simulink model "flightControl"  (R2024a)
settings: Solver=VariableStepAuto  StartTime=0.0  StopTime=25  RelTol=1e-3
settings Model: Creator=Tamir Azaouag  LastModifiedBy=Tamir Azaouag

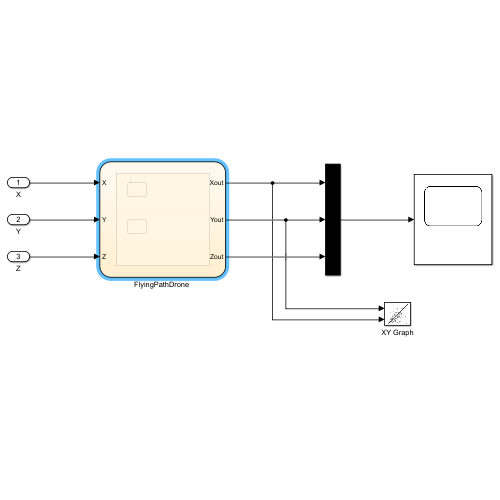
[thumbnail: Simulink's stored preview of the top-level diagram]
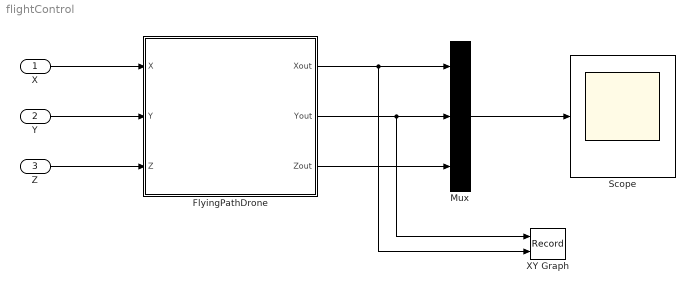
== system flightControl ==
  X : Inport
  Y : Inport  Port=2
  Z : Inport  Port=3
  "FlyingPathDrone " : Stateflow chart  TreatAsAtomicUnit=on
      settings: PortSchema="{\"entries\":[{\"content\":{\"sides\":[{\"content\":{\"connectorIds\":[\"In2\",\"In1\",\"In3\"]},\"type\":\"ConnectorPlacement.EquallySpacedRectSide\",\"uuid\":\"3a0f714e-808a-4da5-be67-da2f18581dd0\"},{\"content\":{\"connectorIds\":[\"Out1\",\"Out2\",\"Out3\"],\"side\":\"RIGHT\"},\"type\":\"ConnectorPlacement.EquallySpacedRectSide\",\"uuid\":\"07aeba56-ef63-4d9e-8974-53c928c3ca5a\"},{\"content\":{\"side\":\"TOP\"},\"type\":\"ConnectorPlacement.EquallySpacedRectSide\",\"uuid\":\"17d58ccf-5bf4-4821-b277-008c533c323a\"}]},\"type\":\"ConnectorPlacement.EquallySpacedConnector\",\"uuid\":\"0ccb1080-62b3-4438-8971-6583531c4324\"}],\"packageUris\":[\"http://schema.mathworks.com/mf0/Connector/R2020b\"],\"version\":\"1.0\"}"
  Mux : Mux  Inputs=3
  Scope : Scope
  XY Graph : Record  FileSettingsInternal="{\"entries\":[{\"content\":{\"excelSettings\":{\"content\":{},\"type\":\"Streamout.ExcelSettings\"}},\"type\":\"Streamout.FileSettingStorage\",\"uuid\":\"\"}],\"packageUris\":[\"http:\\/\\/schema.mathworks.com\\/mf0\\/streamout_blocks\\/R2020a\"],\"version\":\"1.0\"}"  Layout=[1 1]  SignalsInternal="{\"entries\":[{\"content\":{\"signals\":[{\"content\":{\"blockPath\":[],\"dimensions\":[1],\"domain\":\"\",\"lineColor\":\"#a2142f\",\"plots\":[ 1 ],\"port\":1,\"signalID\":1,\"signalName\":\"FlyingPathDrone :2\"},\"type\":\"RecordBlkView.Signal\",\"uuid\":\"\"},{\"content\":{\"blockPath\":[],\"dimensions\":[1],\"domain\":\"\",\"lineColor\":\"#139fff\",\"plots\":[ 1 ],\"port\":2,\"signalID\":2,\"signalName\":\"FlyingPathDrone :1\"},\"type\":\"RecordBlkView.Signal\",\"uuid\":\"\"}]},\"type\":\"RecordBlkView.InputSignals\",\"uuid\":\"\"}],\"packageUris\":[\"http:\\/\\/schema.mathworks.com\\/mf0\\/streamout_blocks\\/R2020a\"],\"version\":\"1.0\"}"  VisualizationBindings="{\"xyplotplugin\":{\"info\":[{\"series\":[{\"bindingParametersList\":[{\"parameter\":\"X-Axis\",\"signalID\":2,\"signalName\":\"FlyingPathDrone :1\"},{\"parameter\":\"Y-Axis\",\"signalID\":1,\"signalName\":\"FlyingPathDrone :2\"}],\"seriesID\":0}],\"subplotID\":1}]}}"  CompatibilityTag=XY
  wires:
  "FlyingPathDrone "/1(Xout) -> XY Graph/2, Mux/1
  "FlyingPathDrone "/2(Yout) -> XY Graph/1, Mux/2
  "FlyingPathDrone "/3(Zout) -> Mux/3
  Mux/1 -> Scope/1
  X/1 -> "FlyingPathDrone "/2(X)
  Y/1 -> "FlyingPathDrone "/1(Y)
  Z/1 -> "FlyingPathDrone "/3(Z)

== stateflow chart flightControl/FlyingPathDrone  ==
  state FlightControl [group]
    state TakeOff
      entry:
      Xout = 0;
      Yout = 0;
      Zout = 0;
      during:
      Zout = Zout - 1
    state Landing
      entry:
      Xout = Xout;
      Yout = Yout;
      Zout = Zout;
      during:
      Zout = Zout + 1
    (default) -> TakeOff
  data: Y input; Xout output; Yout output; Zout output; X input; Z input
